simulink model "fangzhen"  (R2018b)
settings: Solver=ode45  StartTime=0.0  StopTime=10  FixedStep=0.0002  MaxStep=1/5000/25  MinStep=1/5000/100  RelTol=2e-4  EnableMultiTasking=on
libraries: powerlib_meascontrol x6, powerlib x5, simulink x4, powerlib_extras x1
(part 2 of 2)

== system fangzhen/Subsystem2/Subsystem1/SPWM_5 ==
  D : Inport
  Q : Inport  Port=2
  Theta : Inport  Port=3
  Add10 : Sum  Inputs=+-
  Add11 : Sum  Inputs=+-
  Add12 : Sum  Inputs=--
  Add13 : Sum  Inputs=-+
  Add7 : Sum  Inputs=-+
  Add8 : Sum  Inputs=-+
  Add9 : Sum  Inputs=--
  Gain{7..10} (4 alike) : Gain  Gain=sqrt(3)/2
  Gain{3..6} (4 alike) : Gain  Gain=1/2
  Product{8..9,12..13,16..17} (6 alike) : Product  RndMeth=Zero
  Trigonometric Function1 : Trigonometry
  Trigonometric Function4 : Trigonometry  Operator=cos
  a : Outport
  b : Outport  Port=2
  c : Outport  Port=3
  wires:
  Q/1 -> Product17/1, Product12/1, Product9/2
  D/1 -> Product16/1, Product13/1, Product8/2
  Gain10/1 -> Add8/2
  Gain9/1 -> Add13/2
  Gain5/1 -> Add12/1
  Gain8/1 -> Add12/2
  Gain6/1 -> Add13/1
  Add11/1 -> c/1
  Add10/1 -> b/1
  Add7/1 -> a/1
  Add13/1 -> Product17/2
  Add12/1 -> Product16/2
  Product17/1 -> Add11/2
  Product16/1 -> Add11/1
  Add9/1 -> Product12/2
  Add8/1 -> Product13/2
  Product12/1 -> Add10/2
  Product13/1 -> Add10/1
  Gain7/1 -> Add9/2
  Gain4/1 -> Add9/1
  Gain3/1 -> Add8/1
  Product9/1 -> Add7/1
  Trigonometric Function1/1 -> Gain10/1, Gain8/1, Gain6/1, Gain4/1, Product9/1
  Product8/1 -> Add7/2
  Trigonometric Function4/1 -> Gain7/1, Gain9/1, Gain5/1, Gain3/1, Product8/1
  Theta/1 -> Trigonometric Function4/1, Trigonometric Function1/1

== system fangzhen/Subsystem2/Subsystem1/SPWM_7 ==
  D : Inport
  Q : Inport  Port=2
  Theta : Inport  Port=3
  Add10 : Sum  Inputs=+-
  Add11 : Sum  Inputs=+-
  Add12 : Sum  Inputs=--
  Add13 : Sum  Inputs=-+
  Add7 : Sum  Inputs=-+
  Add8 : Sum  Inputs=-+
  Add9 : Sum  Inputs=--
  Gain{7..10} (4 alike) : Gain  Gain=sqrt(3)/2
  Gain{3..6} (4 alike) : Gain  Gain=1/2
  Product{8..9,12..13,16..17} (6 alike) : Product  RndMeth=Zero
  Trigonometric Function1 : Trigonometry
  Trigonometric Function4 : Trigonometry  Operator=cos
  a : Outport
  b : Outport  Port=2
  c : Outport  Port=3
  wires:
  Q/1 -> Product17/1, Product12/1, Product9/2
  D/1 -> Product16/1, Product13/1, Product8/2
  Gain10/1 -> Add8/2
  Gain9/1 -> Add13/2
  Gain5/1 -> Add12/1
  Gain8/1 -> Add12/2
  Gain6/1 -> Add13/1
  Add11/1 -> c/1
  Add10/1 -> b/1
  Add7/1 -> a/1
  Add13/1 -> Product17/2
  Add12/1 -> Product16/2
  Product17/1 -> Add11/2
  Product16/1 -> Add11/1
  Add9/1 -> Product12/2
  Add8/1 -> Product13/2
  Product12/1 -> Add10/2
  Product13/1 -> Add10/1
  Gain7/1 -> Add9/2
  Gain4/1 -> Add9/1
  Gain3/1 -> Add8/1
  Product9/1 -> Add7/1
  Trigonometric Function1/1 -> Gain10/1, Gain8/1, Gain6/1, Gain4/1, Product9/1
  Product8/1 -> Add7/2
  Trigonometric Function4/1 -> Gain7/1, Gain9/1, Gain5/1, Gain3/1, Product8/1
  Theta/1 -> Trigonometric Function4/1, Trigonometric Function1/1

== system fangzhen/Subsystem2/Subsystem1/dq_5 ==
  alpha : Inport
  beta : Inport  Port=2
  theta : Inport  Port=3
  Add4 : Sum
  Add5 : Sum
  Gain1 : Gain  Gain=-1
  Product{,1..3} (4 alike) : Product  RndMeth=Zero
  cos : Trigonometry  Operator=cos
  sin : Trigonometry
  d : Outport
  q : Outport  Port=2
  wires:
  sin/1 -> Product2/1, Product/1
  beta/1 -> Product3/2, Product/2
  cos/1 -> Product3/1, Product1/2
  Add5/1 -> q/1
  theta/1 -> sin/1, cos/1
  Add4/1 -> d/1
  alpha/1 -> Product2/2, Product1/1
  Product1/1 -> Add4/1
  Product/1 -> Add4/2
  Product2/1 -> Gain1/1
  Gain1/1 -> Add5/1
  Product3/1 -> Add5/2

== system fangzhen/Subsystem2/Subsystem1/dq_7 ==
  alpha : Inport
  beta : Inport  Port=2
  theta : Inport  Port=3
  Add4 : Sum
  Add5 : Sum
  Gain1 : Gain  Gain=-1
  Product{,1..3} (4 alike) : Product  RndMeth=Zero
  cos : Trigonometry  Operator=cos
  sin : Trigonometry
  d : Outport
  q : Outport  Port=2
  wires:
  sin/1 -> Product2/1, Product/1
  beta/1 -> Product3/2, Product/2
  cos/1 -> Product3/1, Product1/2
  Add5/1 -> q/1
  theta/1 -> sin/1, cos/1
  Add4/1 -> d/1
  alpha/1 -> Product2/2, Product1/1
  Product1/1 -> Add4/1
  Product/1 -> Add4/2
  Product2/1 -> Gain1/1
  Gain1/1 -> Add5/1
  Product3/1 -> Add5/2

== system fangzhen/Subsystem2/abc//dq current/Clarke1 ==
  In1 : Inport
  In2 : Inport  Port=2
  Constant58 : Constant  Value=3  OutDataTypeStr=double
  Divide : Product  Inputs=*/
  Gain : Gain  Gain=2
  Gain1 : Gain
  Gain2 : Gain
  Sqrt : Sqrt  SaturateOnIntegerOverflow=on
  Sum : Sum
  alpha : Outport
  beta : Outport  Port=2
  wires:
  Divide/1 -> Gain2/1
  Sqrt/1 -> Divide/2
  Constant58/1 -> Sqrt/1
  Sum/1 -> Divide/1
  Gain/1 -> Sum/2
  In1/1 -> Sum/1, Gain1/1
  In2/1 -> Gain/1
  Gain1/1 -> alpha/1
  Gain2/1 -> beta/1

== system fangzhen/Subsystem2/abc//dq current/Park1 ==
  alpha : Inport
  beta : Inport  Port=2
  theta : Inport  Port=3
  Add4 : Sum
  Add5 : Sum
  Gain1 : Gain  Gain=-1
  Product{,1..3} (4 alike) : Product  RndMeth=Zero
  cos : Trigonometry  Operator=cos
  sin : Trigonometry
  d : Outport
  q : Outport  Port=2
  wires:
  Product3/1 -> Add5/2
  Gain1/1 -> Add5/1
  Product2/1 -> Gain1/1
  Product/1 -> Add4/2
  Product1/1 -> Add4/1
  alpha/1 -> Product1/1, Product2/2
  Add4/1 -> d/1
  theta/1 -> cos/1, sin/1
  Add5/1 -> q/1
  cos/1 -> Product1/2, Product3/1
  beta/1 -> Product/2, Product3/2
  sin/1 -> Product/1, Product2/1

== system fangzhen/Subsystem2/angle_evalu/PI-ID3 ==
  err : Inport
  reset : Inport  Port=2
  P : Inport  Port=3
  I : Inport  Port=4
  D : Inport  Port=5
  OV : Inport  Port=6
  Constant1 : Constant  Value=0  OutDataTypeStr=Inherit: Inherit via back propagation
  Constant2 : Constant  Value=25  OutDataTypeStr=Inherit: Inherit via back propagation
  Constant3 : Constant  Value=0  OutDataTypeStr=Inherit: Inherit via back propagation
  Constant5 : Constant  Value=0  OutDataTypeStr=Inherit: Inherit via back propagation
  Logical Operator5 : Logic  AllPortsSameDT=off  OutDataTypeStr=boolean
  Logical Operator6 : Logic  Operator=NOT  AllPortsSameDT=off  OutDataTypeStr=boolean
  Product : Product  RndMeth=Zero
  Product1 : Product  RndMeth=Zero
  Product2 : Product  RndMeth=Zero
  RC filter8 : Subsystem  mask{a=0.4}
      mask prompts: a "Time Constant"
  Saturation : Saturate  UpperLimit=max  LowerLimit=min  LinearizeAsGain=off  ZeroCross=off  OutDataTypeStr=double
  Saturation1 : Saturate  UpperLimit=ermax  LowerLimit=ermin  LinearizeAsGain=off  ZeroCross=off  OutDataTypeStr=double
  Saturation2 : Saturate  UpperLimit=max  LowerLimit=min  LinearizeAsGain=off  ZeroCross=off  OutDataTypeStr=double
  Sum1 : Sum  Inputs=+++
  Sum2 : Sum  Inputs=+-
  Sum4 : Sum
  Switch{1..4} (4 alike) : Switch  Criteria=u2 > Threshold  SaturateOnIntegerOverflow=on  InputSameDT=on
  Unit Delay1 : UnitDelay  SampleTime=-1
  Unit Delay3 : UnitDelay  SampleTime=-1
  out : Outport
  wires:
  Logical Operator6/1 -> Logical Operator5/2
  Logical Operator5/1 -> Switch4/2
  RC filter8/1(y) -> Sum1/3
  Constant3/1 -> Switch3/3
  Switch3/1 -> Switch1/3
  Saturation2/1 -> Switch3/1
  Switch1/1 -> out/1
  OV/1 -> Logical Operator6/1, Switch1/2
  Constant2/1 -> Switch1/1
  Sum1/1 -> Saturation2/1
  Product2/1 -> RC filter8/1(x)
  Unit Delay1/1 -> Sum2/2
  D/1 -> Product2/2
  Sum2/1 -> Product2/1
  Switch4/1 -> Unit Delay3/1
  Unit Delay3/1 -> Sum4/2
  Saturation/1 -> Switch4/1, Sum1/2
  Sum4/1 -> Saturation/1
  Product1/1 -> Sum4/1
  I/1 -> Product1/2
  Product/1 -> Sum1/1
  Saturation1/1 -> Switch2/1
  err/1 -> Saturation1/1
  Constant1/1 -> Switch2/3
  reset/1 -> Logical Operator5/1, Switch3/2, Switch2/2
  Switch2/1 -> Unit Delay1/1, Sum2/1, Product1/1, Product/1
  P/1 -> Product/2
  Constant5/1 -> Switch4/3

== system fangzhen/Subsystem2/angle_evalu/RC filter3 ==
  x : Inport
  Constant2 : Constant  Value=a  OutDataTypeStr=double
  Constant3 : Constant  Value=1-a  OutDataTypeStr=double
  Divide : Product
  Divide1 : Product
  Sum2 : Sum
  Unit Delay2 : UnitDelay  SampleTime=-1
  y : Outport
  wires:
  Unit Delay2/1 -> Divide1/2
  Sum2/1 -> Unit Delay2/1, y/1
  Divide1/1 -> Sum2/2
  Divide/1 -> Sum2/1
  Constant3/1 -> Divide1/1
  Constant2/1 -> Divide/2
  x/1 -> Divide/1

== system fangzhen/Subsystem2/angle_evalu/angle generation ==
  freq : Inport
  Com : simulink/Logic and Bit Operations/Compare To Constant  relop=>=  const=2*pi  OutDataTypeStr=boolean
  Constant3 : Constant  Value=2*pi  OutDataTypeStr=double
  Rem : Math  Operator=rem  SaturateOnIntegerOverflow=on
  Sum11 : Sum
  Switch2 : Switch  Threshold=1
  Unit Delay1 : UnitDelay  SampleTime=-1
  angle_0 : Outport
  wires:
  Unit Delay1/1 -> Sum11/1
  freq/1 -> Sum11/2
  Sum11/1 -> Com/1, Switch2/3, Rem/1
  Switch2/1 -> angle_0/1, Unit Delay1/1
  Com/1 -> Switch2/2
  Rem/1 -> Switch2/1
  Constant3/1 -> Rem/2

== system fangzhen/Subsystem2/Subsystem1/PI-ID5/RC filter8 ==
  x : Inport
  Constant2 : Constant  Value=a  OutDataTypeStr=double
  Constant3 : Constant  Value=1-a  OutDataTypeStr=double
  Divide : Product
  Divide1 : Product
  Sum2 : Sum
  Unit Delay2 : UnitDelay  SampleTime=-1
  y : Outport
  wires:
  Unit Delay2/1 -> Divide1/2
  Sum2/1 -> Unit Delay2/1, y/1
  Divide1/1 -> Sum2/2
  Divide/1 -> Sum2/1
  Constant3/1 -> Divide1/1
  Constant2/1 -> Divide/2
  x/1 -> Divide/1

== system fangzhen/Subsystem2/Subsystem1/PI-ID7/RC filter8 ==
  x : Inport
  Constant2 : Constant  Value=a  OutDataTypeStr=double
  Constant3 : Constant  Value=1-a  OutDataTypeStr=double
  Divide : Product
  Divide1 : Product
  Sum2 : Sum
  Unit Delay2 : UnitDelay  SampleTime=-1
  y : Outport
  wires:
  Unit Delay2/1 -> Divide1/2
  Sum2/1 -> Unit Delay2/1, y/1
  Divide1/1 -> Sum2/2
  Divide/1 -> Sum2/1
  Constant3/1 -> Divide1/1
  Constant2/1 -> Divide/2
  x/1 -> Divide/1

== system fangzhen/Subsystem2/Subsystem1/PI-IQ5/RC filter8 ==
  x : Inport
  Constant2 : Constant  Value=a  OutDataTypeStr=double
  Constant3 : Constant  Value=1-a  OutDataTypeStr=double
  Divide : Product
  Divide1 : Product
  Sum2 : Sum
  Unit Delay2 : UnitDelay  SampleTime=-1
  y : Outport
  wires:
  x/1 -> Divide/1
  Constant2/1 -> Divide/2
  Constant3/1 -> Divide1/1
  Divide/1 -> Sum2/1
  Divide1/1 -> Sum2/2
  Sum2/1 -> y/1, Unit Delay2/1
  Unit Delay2/1 -> Divide1/2

== system fangzhen/Subsystem2/Subsystem1/PI-IQ7/RC filter8 ==
  x : Inport
  Constant2 : Constant  Value=a  OutDataTypeStr=double
  Constant3 : Constant  Value=1-a  OutDataTypeStr=double
  Divide : Product
  Divide1 : Product
  Sum2 : Sum
  Unit Delay2 : UnitDelay  SampleTime=-1
  y : Outport
  wires:
  x/1 -> Divide/1
  Constant2/1 -> Divide/2
  Constant3/1 -> Divide1/1
  Divide/1 -> Sum2/1
  Divide1/1 -> Sum2/2
  Sum2/1 -> y/1, Unit Delay2/1
  Unit Delay2/1 -> Divide1/2

== system fangzhen/Subsystem2/angle_evalu/PI-ID3/RC filter8 ==
  x : Inport
  Constant2 : Constant  Value=a  OutDataTypeStr=double
  Constant3 : Constant  Value=1-a  OutDataTypeStr=double
  Divide : Product
  Divide1 : Product
  Sum2 : Sum
  Unit Delay2 : UnitDelay  SampleTime=-1
  y : Outport
  wires:
  Unit Delay2/1 -> Divide1/2
  Sum2/1 -> Unit Delay2/1, y/1
  Divide1/1 -> Sum2/2
  Divide/1 -> Sum2/1
  Constant3/1 -> Divide1/1
  Constant2/1 -> Divide/2
  x/1 -> Divide/1
